simulink model "l512_devel_pps"  (R2012b)
settings: Solver=ode45  StartTime=0.0  StopTime=15000  RelTol=1e-3
undefined symbols (not defined in the file): sfp
libraries: xbsIndex_r4 x6414, casper_library_misc x268, casper_library_delays x134, xps_library x12, simulink x1, gavrt_library x1, xbsReplacements_r4 x1
(part 13 of 67)

== system l512_devel_pps/fft/f3/rms_mon_4b ==
  note: Value on vin
      | aligned with
      | first sample on
      | din captured
  note: Number of valid
      | data samples to
      | skip after trigger
      | before starting
      | capture
  note: Number of
      | bytes in
      | buffer and
      | done bit
  note: Offset in vector
      | from first element
      | captured, used
      | during circular capture
  note: ctrl:
      | bit0: Put a posedge here
      |         to enable a new capture.
      | bit1: ignore external trigger
      |         and trigger immediately.
      | bit2: ignore external write
      |         enable and capture on
      |         every FPGA clock.
      | bit3: continuously capture
      |         data until we get an
      |         external stop command.
  note: Delay start
      | of capture
  note: Generate stop
      | when in circular
      | capture mode
  din : Inport
  we : Inport  Port=2
  trig : Inport  Port=3
  add_del : xbsIndex_r4/Delay  rst=off  infoeditControl=Selection of Reset will increase slice count due to use of real FFs and instead of SRLs  en=off  latency=1  dbl_ovrd=off  reg_retiming=on  block_type=delay
      settings: block_version=11.4
  add_gen : Subsystem  AncestorBlock=casper_library_scopes/snapshot/add_gen  mask{counter_size=12+0+1, increment=1, nsamples=12, burst_size=0, use_dsp48=off}
      mask prompts: counter_size "Address counter size (2^?)"; increment "Address counter increment"; nsamples "Number of samples (2^?)"; burst_size "Burst size (2^?)"; use_dsp48 "dsp48 counter/s"
      mask init:
      | set_param(gcb,'LinkStatus','inactive');
      | if strcmp(use_dsp48,'on'),
      |     set_param([gcb,'/add_gen'],'implementation','DSP48');
      | else
      |     set_param([gcb,'/add_gen'],'implementation','Fabric');
      | end
  basic_ctrl : Subsystem  AncestorBlock=casper_library_scopes/snapshot/basic_ctrl  mask{dram=off, data_width=8}
      mask prompts: data_width "data width"
      mask init:
      | set_param(gcb,'LinkStatus','inactive');
      | set_param([gcb,'/dram_munge'], 'dram', dram);
  bram : Subsystem  Tag=xps:bram  AncestorBlock=xps_library/Shared BRAM  mask{arith_type=Unsigned, addr_width=12, data_width=8, reg_prim_output=on, reg_core_output=on, optimization=Minimum_Area, data_bin_pt=0, init_vals=[0:2^10-1], sample_rate=1}
      mask prompts: arith_type "Output Data Type"; addr_width "Address width"; data_width "Data Width"; reg_prim_output "Register Primitive Output"; reg_core_output "Register Core Output"; data_bin_pt "Data Binary Point"; init_vals "Initial values (simulation only)"; sample_rate "Sample rate"
      mask init:
      | shared_bram_mask;
      mask TypeOptions arith_type: Unsigned | Signed  (2's comp)
      mask TypeOptions data_width: 8 | 16 | 32 | 64 | 128
      mask TypeOptions optimization: Minimum_Area | Low_Power
  cast : xbsIndex_r4/Convert  gui_display_data_type=Fixed-point  arith_type=Unsigned  n_bits=8  bin_pt=0  float_type=Single  exp_bits=8  fraction_bits=24  quantization=Truncate  overflow=Wrap  en=off  latency=0  dbl_ovrd=off  pipeline=off  block_type=convert
      settings: block_version=11.4
  circular_capture : casper_library_misc/info_block  Tag=casper:info  info=off
  const0 : Constant  Value=0
  ctrl : Subsystem  Tag=xps:sw_reg  AncestorBlock=xps_library/software register  mask{numios=1, io_dir=From Processor, io_delay=0, sample_period=1, name1=reg, bitwidth1=32, arith_type1=Unsigned, bin_pt1=0}
      mask prompts: numios "Num I/Os"; io_dir "I/O direction"; io_delay "I/O delay"; sample_period "Sample period"; name1 "Name"; bitwidth1 "Bitwidth"; arith_type1 "Type"; bin_pt1 "Binary pt"
      mask init:
      | swreg_init(gcb);
      mask Callback numios: t = timer('StartDelay', 0.1); t.TimerFcn = {@swreg_cb, gcb}; start(t);
      mask TypeOptions io_dir: To Processor | From Processor
      mask Callback io_dir:
      | a = get_param(gcb, 'MaskEnables');
      | if strcmp(get_param(gcb, 'io_dir'), 'To Processor'),
      | a(4) = {'off'};
      | else
      | a(4) = {'on'};
      | end
      | set_param(gcb, 'MaskEnables', a);
      mask TypeOptions arith_type1: Unsigned | Signed  (2's comp) | Boolean
      mask Callback arith_type1:
      | a = get_param(gcb, 'MaskEnables');
      | if strcmp(get_param(gcb, 'arith_type1'), 'Boolean'),
      | set_param(gcb, 'bitwidth1', '1');
      | set_param(gcb, 'bin_pt1', '0');
      | a(6) = {'off'};
      | a(8) = {'off'};
      | else
      | a(6) = {'on'};
      | a(8) = {'on'};
      | end
      | set_param(gcb, 'MaskEnables', a);
  dat_del : xbsIndex_r4/Delay  rst=off  infoeditControl=Selection of Reset will increase slice count due to use of real FFs and instead of SRLs  en=off  latency=1  dbl_ovrd=off  reg_retiming=on  block_type=delay
      settings: block_version=11.4
  data_width : casper_library_misc/info_block  Tag=casper:info  info=8
  dram_clock : casper_library_misc/info_block  Tag=casper:info  info=200
  dram_dimm : casper_library_misc/info_block  Tag=casper:info  info=1
  extra_value : casper_library_misc/info_block  Tag=casper:info  info=off
  g_tr_en_cnt : Terminator
  gbram : Terminator
  gstatus : Terminator
  gval : Terminator
  length : casper_library_misc/info_block  Tag=casper:info  info=4096
  never : xbsIndex_r4/Constant  const=0  gui_display_data_type=Fixed-point  arith_type=Boolean  n_bits=16  bin_pt=14  preci_type=Single  exp_width=8  frac_width=24  explicit_period=on  period=1  equ=P=C  opselect=C  inp2=PCIN>>17  opr=+  inp1=P  carry=CIN  dbl_ovrd=off  block_type=constant
  ri : xbsIndex_r4/Reinterpret  force_arith_type=on  arith_type=Unsigned  force_bin_pt=on  bin_pt=0  block_type=reinterpret
      settings: infoedit="Changes signal type without altering the binary representation.   You can changed the signal between signed and unsigned, and relocate the binary point.<br><br>Hardware notes: In hardware this block costs nothing.<br><br>Example:  Suppose the input is 6 bits wide, signed, with 2 fractional bits, and the output is forced to unsigned with 0 fractional bits.  Then an input of -2.0 (1110.00 in binary 2's complement) becomes an output of 56 (111000 in binary)."
  start_offset : casper_library_misc/info_block  Tag=casper:info  info=off
  status : Subsystem  Tag=xps:sw_reg  AncestorBlock=xps_library/software register  mask{numios=1, io_dir=To Processor, io_delay=0, sample_period=1, name1=reg, bitwidth1=32, arith_type1=Unsigned, bin_pt1=0}
      mask prompts: numios "Num I/Os"; io_dir "I/O direction"; io_delay "I/O delay"; sample_period "Sample period"; name1 "Name"; bitwidth1 "Bitwidth"; arith_type1 "Type"; bin_pt1 "Binary pt"
      mask init:
      | swreg_init(gcb);
      mask Callback numios: t = timer('StartDelay', 0.1); t.TimerFcn = {@swreg_cb, gcb}; start(t);
      mask TypeOptions io_dir: To Processor | From Processor
      mask Callback io_dir:
      | a = get_param(gcb, 'MaskEnables');
      | if strcmp(get_param(gcb, 'io_dir'), 'To Processor'),
      | a(4) = {'off'};
      | else
      | a(4) = {'on'};
      | end
      | set_param(gcb, 'MaskEnables', a);
      mask TypeOptions arith_type1: Unsigned | Signed  (2's comp) | Boolean
      mask Callback arith_type1:
      | a = get_param(gcb, 'MaskEnables');
      | if strcmp(get_param(gcb, 'arith_type1'), 'Boolean'),
      | set_param(gcb, 'bitwidth1', '1');
      | set_param(gcb, 'bin_pt1', '0');
      | a(6) = {'off'};
      | a(8) = {'off'};
      | else
      | a(6) = {'on'};
      | a(8) = {'on'};
      | end
      | set_param(gcb, 'MaskEnables', a);
  storage : casper_library_misc/info_block  Tag=casper:info  info=bram
  use_dsp48 : casper_library_misc/info_block  Tag=casper:info  info=off
  vin_const : xbsIndex_r4/Constant  const=0  gui_display_data_type=Fixed-point  arith_type=Boolean  n_bits=16  bin_pt=14  preci_type=Single  exp_width=8  frac_width=24  explicit_period=on  period=1  equ=P=C  opselect=C  inp2=PCIN>>17  opr=+  inp1=P  carry=CIN  dbl_ovrd=off  block_type=constant
      settings: block_version=11.4
  we_del : xbsIndex_r4/Delay  rst=off  infoeditControl=Selection of Reset will increase slice count due to use of real FFs and instead of SRLs  en=off  latency=1  dbl_ovrd=off  reg_retiming=on  block_type=delay
      settings: block_version=11.4
  wires:
  bram/1(data_out) -> gbram/1
  we_del/1 -> bram/3(we)
  dat_del/1 -> bram/2(data_in)
  add_del/1 -> bram/1(addr)
  add_gen/4(we_o) -> we_del/1
  add_gen/3(dout) -> dat_del/1
  add_gen/2(add) -> add_del/1
  add_gen/6(en_cnt) -> g_tr_en_cnt/1
  add_gen/1(vout) -> gval/1
  vin_const/1 -> basic_ctrl/1(vin)
  status/1(sim_out) -> gstatus/1
  add_gen/5(status) -> status/1(out_reg)
  basic_ctrl/6(init) -> add_gen/6(init)
  basic_ctrl/5(stop) -> add_gen/5(cont)
  basic_ctrl/4(go) -> add_gen/4(go)
  basic_ctrl/3(we_o) -> add_gen/3(we)
  basic_ctrl/2(dout) -> add_gen/2(din)
  basic_ctrl/1(vout) -> add_gen/1(vin)
  ctrl/1(in_reg) -> basic_ctrl/5(ctrl)
  const0/1 -> ctrl/1(sim_reg)
  never/1 -> basic_ctrl/6(stopi)
  trig/1 -> basic_ctrl/4(trig)
  we/1 -> basic_ctrl/3(we)
  cast/1 -> basic_ctrl/2(din)
  ri/1 -> cast/1
  din/1 -> ri/1

== system l512_devel_pps/fft/f3/spec0 ==
  sync_in : Inport
  pps_in : Inport  Port=2
  d_in : Inport  Port=3
  bitsel : Inport  Port=4
  acc_len : Inport  Port=5
  Delay1 : xbsIndex_r4/Delay  rst=off  infoeditControl=Selection of Reset will increase slice count due to use of real FFs and instead of SRLs  en=off  latency=4  dbl_ovrd=off  reg_retiming=off  block_type=delay
  Delay2 : xbsIndex_r4/Delay  rst=off  infoeditControl=Selection of Reset will increase slice count due to use of real FFs and instead of SRLs  en=off  latency=2  dbl_ovrd=off  reg_retiming=off  block_type=delay
  Delay6 : xbsIndex_r4/Delay  rst=off  infoeditControl=Selection of Reset will increase slice count due to use of real FFs and instead of SRLs  en=off  latency=2  dbl_ovrd=off  reg_retiming=off  block_type=delay
  edge_detect2 : casper_library_misc/edge_detect  edge=Rising  polarity=Active High  x_in=[0 0.08 0.08 0.16 0.16 0.24 0.24 0.32 0.32 0.4]  y_in="[-1 -1  1  1  1  1  1  1  1  1]"  x_out=[0.6 0.68 0.68 0.76 0.76 0.84 0.84 0.92 0.92 1]  y_out="[-1 -1  1  1 -1 -1 -1 -1 -1 -1]"
  pipeline4 : Subsystem  AncestorBlock=casper_library_delays/pipeline  mask(pipeline){latency=1}
      mask help:
      | An explicitly laid-out delay line to avoid mapping to SRL16s
      | for use in pipelining to help achieve timing closure.
      mask init:
      | pipeline_init(gcb,'latency',latency);
      settings: AttributesFormatString=Latency = %<latency>
      mask Display:
      | port_label('input', 1, 'd');
      | port_label('output', 1, 'q');
      | disp(['Z^-', num2str(latency)]);
  pipeline5 : Subsystem  AncestorBlock=casper_library_delays/pipeline  mask(pipeline){latency=1}
      mask help:
      | An explicitly laid-out delay line to avoid mapping to SRL16s
      | for use in pipelining to help achieve timing closure.
      mask init:
      | pipeline_init(gcb,'latency',latency);
      settings: AttributesFormatString=Latency = %<latency>
      mask Display:
      | port_label('input', 1, 'd');
      | port_label('output', 1, 'q');
      | disp(['Z^-', num2str(latency)]);
  pipeline6 : Subsystem  AncestorBlock=casper_library_delays/pipeline  mask(pipeline){latency=1}
      mask help:
      | An explicitly laid-out delay line to avoid mapping to SRL16s
      | for use in pipelining to help achieve timing closure.
      mask init:
      | pipeline_init(gcb,'latency',latency);
      settings: AttributesFormatString=Latency = %<latency>
      mask Display:
      | port_label('input', 1, 'd');
      | port_label('output', 1, 'q');
      | disp(['Z^-', num2str(latency)]);
  power_dsp48e3 : casper_library_misc/power_dsp48e  bitwidth=18
  rq : Subsystem
  snap : Subsystem  mask{vec_bits=12}
      mask prompts: vec_bits "Vector length (2^N)"
  sync_delay : casper_library_delays/sync_delay  DelayLen=10
  vacc_pps : Subsystem  mask{n_fft=12}
      mask prompts: n_fft "Length of FFT (2^N)?"
  vacc_zeroer1 : Subsystem  mask{nbits=13, bw=16}
      mask prompts: nbits "FFT length (2^N)?"; bw "bitwidth in"
      mask help: FFT length is full length of FFT. The second half will be blanked.
  new_acc : Outport
  wires:
  vacc_pps/2(d_out) -> pipeline4/1(d)
  vacc_zeroer1/1(sync_out) -> vacc_pps/1(sync_in)
  sync_delay/1 -> vacc_pps/2(pps_in)
  pps_in/1 -> sync_delay/1
  power_dsp48e3/1 -> rq/2(d_in)
  pipeline6/1(q) -> edge_detect2/1
  bitsel/1 -> rq/3(bitsel)
  vacc_zeroer1/2(d_out) -> vacc_pps/4(d_in)
  d_in/1 -> power_dsp48e3/1
  sync_in/1 -> Delay1/1
  rq/2(d_out) -> vacc_zeroer1/2(d_in)
  Delay1/1 -> rq/1(sync_in)
  Delay6/1 -> snap/2(data_valid)
  acc_len/1 -> vacc_pps/3(acc_len)
  edge_detect2/1 -> snap/1(new_acc), new_acc/1
  pipeline4/1(q) -> Delay2/1
  Delay2/1 -> snap/3(xx_in)
  vacc_pps/1(valid_out) -> pipeline5/1(d), pipeline6/1(d)
  rq/1(sync_out) -> vacc_zeroer1/1(sync_in)
  pipeline5/1(q) -> Delay6/1

== system l512_devel_pps/fft/f3/spec1 ==
  sync_in : Inport
  pps_in : Inport  Port=2
  d_in : Inport  Port=3
  bitsel : Inport  Port=4
  acc_len : Inport  Port=5
  Delay1 : xbsIndex_r4/Delay  rst=off  infoeditControl=Selection of Reset will increase slice count due to use of real FFs and instead of SRLs  en=off  latency=4  dbl_ovrd=off  reg_retiming=off  block_type=delay
  Delay2 : xbsIndex_r4/Delay  rst=off  infoeditControl=Selection of Reset will increase slice count due to use of real FFs and instead of SRLs  en=off  latency=2  dbl_ovrd=off  reg_retiming=off  block_type=delay
  Delay6 : xbsIndex_r4/Delay  rst=off  infoeditControl=Selection of Reset will increase slice count due to use of real FFs and instead of SRLs  en=off  latency=2  dbl_ovrd=off  reg_retiming=off  block_type=delay
  edge_detect2 : casper_library_misc/edge_detect  edge=Rising  polarity=Active High  x_in=[0 0.08 0.08 0.16 0.16 0.24 0.24 0.32 0.32 0.4]  y_in="[-1 -1  1  1  1  1  1  1  1  1]"  x_out=[0.6 0.68 0.68 0.76 0.76 0.84 0.84 0.92 0.92 1]  y_out="[-1 -1  1  1 -1 -1 -1 -1 -1 -1]"
  pipeline4 : Subsystem  AncestorBlock=casper_library_delays/pipeline  mask(pipeline){latency=1}
      mask help:
      | An explicitly laid-out delay line to avoid mapping to SRL16s
      | for use in pipelining to help achieve timing closure.
      mask init:
      | pipeline_init(gcb,'latency',latency);
      settings: AttributesFormatString=Latency = %<latency>
      mask Display:
      | port_label('input', 1, 'd');
      | port_label('output', 1, 'q');
      | disp(['Z^-', num2str(latency)]);
  pipeline5 : Subsystem  AncestorBlock=casper_library_delays/pipeline  mask(pipeline){latency=1}
      mask help:
      | An explicitly laid-out delay line to avoid mapping to SRL16s
      | for use in pipelining to help achieve timing closure.
      mask init:
      | pipeline_init(gcb,'latency',latency);
      settings: AttributesFormatString=Latency = %<latency>
      mask Display:
      | port_label('input', 1, 'd');
      | port_label('output', 1, 'q');
      | disp(['Z^-', num2str(latency)]);
  pipeline6 : Subsystem  AncestorBlock=casper_library_delays/pipeline  mask(pipeline){latency=1}
      mask help:
      | An explicitly laid-out delay line to avoid mapping to SRL16s
      | for use in pipelining to help achieve timing closure.
      mask init:
      | pipeline_init(gcb,'latency',latency);
      settings: AttributesFormatString=Latency = %<latency>
      mask Display:
      | port_label('input', 1, 'd');
      | port_label('output', 1, 'q');
      | disp(['Z^-', num2str(latency)]);
  power_dsp48e3 : casper_library_misc/power_dsp48e  bitwidth=18
  rq : Subsystem
  snap : Subsystem  mask{vec_bits=12}
      mask prompts: vec_bits "Vector length (2^N)"
  sync_delay : casper_library_delays/sync_delay  DelayLen=10
  vacc_pps : Subsystem  mask{n_fft=12}
      mask prompts: n_fft "Length of FFT (2^N)?"
  vacc_zeroer1 : Subsystem  mask{nbits=13, bw=16}
      mask prompts: nbits "FFT length (2^N)?"; bw "bitwidth in"
      mask help: FFT length is full length of FFT. The second half will be blanked.
  new_acc : Outport
  wires:
  pipeline5/1(q) -> Delay6/1
  rq/1(sync_out) -> vacc_zeroer1/1(sync_in)
  vacc_pps/1(valid_out) -> pipeline6/1(d), pipeline5/1(d)
  Delay2/1 -> snap/3(xx_in)
  pipeline4/1(q) -> Delay2/1
  edge_detect2/1 -> new_acc/1, snap/1(new_acc)
  acc_len/1 -> vacc_pps/3(acc_len)
  Delay6/1 -> snap/2(data_valid)
  Delay1/1 -> rq/1(sync_in)
  rq/2(d_out) -> vacc_zeroer1/2(d_in)
  sync_in/1 -> Delay1/1
  d_in/1 -> power_dsp48e3/1
  vacc_zeroer1/2(d_out) -> vacc_pps/4(d_in)
  bitsel/1 -> rq/3(bitsel)
  pipeline6/1(q) -> edge_detect2/1
  power_dsp48e3/1 -> rq/2(d_in)
  pps_in/1 -> sync_delay/1
  sync_delay/1 -> vacc_pps/2(pps_in)
  vacc_zeroer1/1(sync_out) -> vacc_pps/1(sync_in)
  vacc_pps/2(d_out) -> pipeline4/1(d)

== system l512_devel_pps/fft/f3/spec2 ==
  sync_in : Inport
  pps_in : Inport  Port=2
  d_in : Inport  Port=3
  bitsel : Inport  Port=4
  acc_len : Inport  Port=5
  Delay1 : xbsIndex_r4/Delay  rst=off  infoeditControl=Selection of Reset will increase slice count due to use of real FFs and instead of SRLs  en=off  latency=4  dbl_ovrd=off  reg_retiming=off  block_type=delay
  Delay2 : xbsIndex_r4/Delay  rst=off  infoeditControl=Selection of Reset will increase slice count due to use of real FFs and instead of SRLs  en=off  latency=2  dbl_ovrd=off  reg_retiming=off  block_type=delay
  Delay6 : xbsIndex_r4/Delay  rst=off  infoeditControl=Selection of Reset will increase slice count due to use of real FFs and instead of SRLs  en=off  latency=2  dbl_ovrd=off  reg_retiming=off  block_type=delay
  edge_detect2 : casper_library_misc/edge_detect  edge=Rising  polarity=Active High  x_in=[0 0.08 0.08 0.16 0.16 0.24 0.24 0.32 0.32 0.4]  y_in="[-1 -1  1  1  1  1  1  1  1  1]"  x_out=[0.6 0.68 0.68 0.76 0.76 0.84 0.84 0.92 0.92 1]  y_out="[-1 -1  1  1 -1 -1 -1 -1 -1 -1]"
  pipeline4 : Subsystem  AncestorBlock=casper_library_delays/pipeline  mask(pipeline){latency=1}
      mask help:
      | An explicitly laid-out delay line to avoid mapping to SRL16s
      | for use in pipelining to help achieve timing closure.
      mask init:
      | pipeline_init(gcb,'latency',latency);
      settings: AttributesFormatString=Latency = %<latency>
      mask Display:
      | port_label('input', 1, 'd');
      | port_label('output', 1, 'q');
      | disp(['Z^-', num2str(latency)]);
  pipeline5 : Subsystem  AncestorBlock=casper_library_delays/pipeline  mask(pipeline){latency=1}
      mask help:
      | An explicitly laid-out delay line to avoid mapping to SRL16s
      | for use in pipelining to help achieve timing closure.
      mask init:
      | pipeline_init(gcb,'latency',latency);
      settings: AttributesFormatString=Latency = %<latency>
      mask Display:
      | port_label('input', 1, 'd');
      | port_label('output', 1, 'q');
      | disp(['Z^-', num2str(latency)]);
  pipeline6 : Subsystem  AncestorBlock=casper_library_delays/pipeline  mask(pipeline){latency=1}
      mask help:
      | An explicitly laid-out delay line to avoid mapping to SRL16s
      | for use in pipelining to help achieve timing closure.
      mask init:
      | pipeline_init(gcb,'latency',latency);
      settings: AttributesFormatString=Latency = %<latency>
      mask Display:
      | port_label('input', 1, 'd');
      | port_label('output', 1, 'q');
      | disp(['Z^-', num2str(latency)]);
  power_dsp48e3 : casper_library_misc/power_dsp48e  bitwidth=18
  rq : Subsystem
  snap : Subsystem  mask{vec_bits=12}
      mask prompts: vec_bits "Vector length (2^N)"
  sync_delay : casper_library_delays/sync_delay  DelayLen=10
  vacc_pps : Subsystem  mask{n_fft=12}
      mask prompts: n_fft "Length of FFT (2^N)?"
  vacc_zeroer1 : Subsystem  mask{nbits=13, bw=16}
      mask prompts: nbits "FFT length (2^N)?"; bw "bitwidth in"
      mask help: FFT length is full length of FFT. The second half will be blanked.
  new_acc : Outport
  wires:
  vacc_pps/2(d_out) -> pipeline4/1(d)
  vacc_zeroer1/1(sync_out) -> vacc_pps/1(sync_in)
  sync_delay/1 -> vacc_pps/2(pps_in)
  pps_in/1 -> sync_delay/1
  power_dsp48e3/1 -> rq/2(d_in)
  pipeline6/1(q) -> edge_detect2/1
  bitsel/1 -> rq/3(bitsel)
  vacc_zeroer1/2(d_out) -> vacc_pps/4(d_in)
  d_in/1 -> power_dsp48e3/1
  sync_in/1 -> Delay1/1
  rq/2(d_out) -> vacc_zeroer1/2(d_in)
  Delay1/1 -> rq/1(sync_in)
  Delay6/1 -> snap/2(data_valid)
  acc_len/1 -> vacc_pps/3(acc_len)
  edge_detect2/1 -> snap/1(new_acc), new_acc/1
  pipeline4/1(q) -> Delay2/1
  Delay2/1 -> snap/3(xx_in)
  vacc_pps/1(valid_out) -> pipeline5/1(d), pipeline6/1(d)
  rq/1(sync_out) -> vacc_zeroer1/1(sync_in)
  pipeline5/1(q) -> Delay6/1

== system l512_devel_pps/fft/f3/spec3 ==
  sync_in : Inport
  pps_in : Inport  Port=2
  d_in : Inport  Port=3
  bitsel : Inport  Port=4
  acc_len : Inport  Port=5
  Delay1 : xbsIndex_r4/Delay  rst=off  infoeditControl=Selection of Reset will increase slice count due to use of real FFs and instead of SRLs  en=off  latency=4  dbl_ovrd=off  reg_retiming=off  block_type=delay
  Delay2 : xbsIndex_r4/Delay  rst=off  infoeditControl=Selection of Reset will increase slice count due to use of real FFs and instead of SRLs  en=off  latency=2  dbl_ovrd=off  reg_retiming=off  block_type=delay
  Delay6 : xbsIndex_r4/Delay  rst=off  infoeditControl=Selection of Reset will increase slice count due to use of real FFs and instead of SRLs  en=off  latency=2  dbl_ovrd=off  reg_retiming=off  block_type=delay
  edge_detect2 : casper_library_misc/edge_detect  edge=Rising  polarity=Active High  x_in=[0 0.08 0.08 0.16 0.16 0.24 0.24 0.32 0.32 0.4]  y_in="[-1 -1  1  1  1  1  1  1  1  1]"  x_out=[0.6 0.68 0.68 0.76 0.76 0.84 0.84 0.92 0.92 1]  y_out="[-1 -1  1  1 -1 -1 -1 -1 -1 -1]"
  pipeline4 : Subsystem  AncestorBlock=casper_library_delays/pipeline  mask(pipeline){latency=1}
      mask help:
      | An explicitly laid-out delay line to avoid mapping to SRL16s
      | for use in pipelining to help achieve timing closure.
      mask init:
      | pipeline_init(gcb,'latency',latency);
      settings: AttributesFormatString=Latency = %<latency>
      mask Display:
      | port_label('input', 1, 'd');
      | port_label('output', 1, 'q');
      | disp(['Z^-', num2str(latency)]);
  pipeline5 : Subsystem  AncestorBlock=casper_library_delays/pipeline  mask(pipeline){latency=1}
      mask help:
      | An explicitly laid-out delay line to avoid mapping to SRL16s
      | for use in pipelining to help achieve timing closure.
      mask init:
      | pipeline_init(gcb,'latency',latency);
      settings: AttributesFormatString=Latency = %<latency>
      mask Display:
      | port_label('input', 1, 'd');
      | port_label('output', 1, 'q');
      | disp(['Z^-', num2str(latency)]);
  pipeline6 : Subsystem  AncestorBlock=casper_library_delays/pipeline  mask(pipeline){latency=1}
      mask help:
      | An explicitly laid-out delay line to avoid mapping to SRL16s
      | for use in pipelining to help achieve timing closure.
      mask init:
      | pipeline_init(gcb,'latency',latency);
      settings: AttributesFormatString=Latency = %<latency>
      mask Display:
      | port_label('input', 1, 'd');
      | port_label('output', 1, 'q');
      | disp(['Z^-', num2str(latency)]);
  power_dsp48e3 : casper_library_misc/power_dsp48e  bitwidth=18
  rq : Subsystem
  snap : Subsystem  mask{vec_bits=12}
      mask prompts: vec_bits "Vector length (2^N)"
  sync_delay : casper_library_delays/sync_delay  DelayLen=10
  vacc_pps : Subsystem  mask{n_fft=12}
      mask prompts: n_fft "Length of FFT (2^N)?"
  vacc_zeroer1 : Subsystem  mask{nbits=13, bw=16}
      mask prompts: nbits "FFT length (2^N)?"; bw "bitwidth in"
      mask help: FFT length is full length of FFT. The second half will be blanked.
  new_acc : Outport
  wires:
  pipeline5/1(q) -> Delay6/1
  rq/1(sync_out) -> vacc_zeroer1/1(sync_in)
  vacc_pps/1(valid_out) -> pipeline6/1(d), pipeline5/1(d)
  Delay2/1 -> snap/3(xx_in)
  pipeline4/1(q) -> Delay2/1
  edge_detect2/1 -> new_acc/1, snap/1(new_acc)
  acc_len/1 -> vacc_pps/3(acc_len)
  Delay6/1 -> snap/2(data_valid)
  Delay1/1 -> rq/1(sync_in)
  rq/2(d_out) -> vacc_zeroer1/2(d_in)
  sync_in/1 -> Delay1/1
  d_in/1 -> power_dsp48e3/1
  vacc_zeroer1/2(d_out) -> vacc_pps/4(d_in)
  bitsel/1 -> rq/3(bitsel)
  pipeline6/1(q) -> edge_detect2/1
  power_dsp48e3/1 -> rq/2(d_in)
  pps_in/1 -> sync_delay/1
  sync_delay/1 -> vacc_pps/2(pps_in)
  vacc_zeroer1/1(sync_out) -> vacc_pps/1(sync_in)
  vacc_pps/2(d_out) -> pipeline4/1(d)

== system l512_devel_pps/fft/f3/spec4 ==
  sync_in : Inport
  pps_in : Inport  Port=2
  d_in : Inport  Port=3
  bitsel : Inport  Port=4
  acc_len : Inport  Port=5
  Delay1 : xbsIndex_r4/Delay  rst=off  infoeditControl=Selection of Reset will increase slice count due to use of real FFs and instead of SRLs  en=off  latency=4  dbl_ovrd=off  reg_retiming=off  block_type=delay
  Delay2 : xbsIndex_r4/Delay  rst=off  infoeditControl=Selection of Reset will increase slice count due to use of real FFs and instead of SRLs  en=off  latency=2  dbl_ovrd=off  reg_retiming=off  block_type=delay
  Delay6 : xbsIndex_r4/Delay  rst=off  infoeditControl=Selection of Reset will increase slice count due to use of real FFs and instead of SRLs  en=off  latency=2  dbl_ovrd=off  reg_retiming=off  block_type=delay
  edge_detect2 : casper_library_misc/edge_detect  edge=Rising  polarity=Active High  x_in=[0 0.08 0.08 0.16 0.16 0.24 0.24 0.32 0.32 0.4]  y_in="[-1 -1  1  1  1  1  1  1  1  1]"  x_out=[0.6 0.68 0.68 0.76 0.76 0.84 0.84 0.92 0.92 1]  y_out="[-1 -1  1  1 -1 -1 -1 -1 -1 -1]"
  pipeline4 : Subsystem  AncestorBlock=casper_library_delays/pipeline  mask(pipeline){latency=1}
      mask help:
      | An explicitly laid-out delay line to avoid mapping to SRL16s
      | for use in pipelining to help achieve timing closure.
      mask init:
      | pipeline_init(gcb,'latency',latency);
      settings: AttributesFormatString=Latency = %<latency>
      mask Display:
      | port_label('input', 1, 'd');
      | port_label('output', 1, 'q');
      | disp(['Z^-', num2str(latency)]);
  pipeline5 : Subsystem  AncestorBlock=casper_library_delays/pipeline  mask(pipeline){latency=1}
      mask help:
      | An explicitly laid-out delay line to avoid mapping to SRL16s
      | for use in pipelining to help achieve timing closure.
      mask init:
      | pipeline_init(gcb,'latency',latency);
      settings: AttributesFormatString=Latency = %<latency>
      mask Display:
      | port_label('input', 1, 'd');
      | port_label('output', 1, 'q');
      | disp(['Z^-', num2str(latency)]);
  pipeline6 : Subsystem  AncestorBlock=casper_library_delays/pipeline  mask(pipeline){latency=1}
      mask help:
      | An explicitly laid-out delay line to avoid mapping to SRL16s
      | for use in pipelining to help achieve timing closure.
      mask init:
      | pipeline_init(gcb,'latency',latency);
      settings: AttributesFormatString=Latency = %<latency>
      mask Display:
      | port_label('input', 1, 'd');
      | port_label('output', 1, 'q');
      | disp(['Z^-', num2str(latency)]);
  power_dsp48e3 : casper_library_misc/power_dsp48e  bitwidth=18
  rq : Subsystem
  snap : Subsystem  mask{vec_bits=12}
      mask prompts: vec_bits "Vector length (2^N)"
  sync_delay : casper_library_delays/sync_delay  DelayLen=10
  vacc_pps : Subsystem  mask{n_fft=12}
      mask prompts: n_fft "Length of FFT (2^N)?"
  vacc_zeroer1 : Subsystem  mask{nbits=13, bw=16}
      mask prompts: nbits "FFT length (2^N)?"; bw "bitwidth in"
      mask help: FFT length is full length of FFT. The second half will be blanked.
  new_acc : Outport
  wires:
  vacc_pps/2(d_out) -> pipeline4/1(d)
  vacc_zeroer1/1(sync_out) -> vacc_pps/1(sync_in)
  sync_delay/1 -> vacc_pps/2(pps_in)
  pps_in/1 -> sync_delay/1
  power_dsp48e3/1 -> rq/2(d_in)
  pipeline6/1(q) -> edge_detect2/1
  bitsel/1 -> rq/3(bitsel)
  vacc_zeroer1/2(d_out) -> vacc_pps/4(d_in)
  d_in/1 -> power_dsp48e3/1
  sync_in/1 -> Delay1/1
  rq/2(d_out) -> vacc_zeroer1/2(d_in)
  Delay1/1 -> rq/1(sync_in)
  Delay6/1 -> snap/2(data_valid)
  acc_len/1 -> vacc_pps/3(acc_len)
  edge_detect2/1 -> snap/1(new_acc), new_acc/1
  pipeline4/1(q) -> Delay2/1
  Delay2/1 -> snap/3(xx_in)
  vacc_pps/1(valid_out) -> pipeline5/1(d), pipeline6/1(d)
  rq/1(sync_out) -> vacc_zeroer1/1(sync_in)
  pipeline5/1(q) -> Delay6/1

== system l512_devel_pps/fft/f3/spec5 ==
  sync_in : Inport
  pps_in : Inport  Port=2
  d_in : Inport  Port=3
  bitsel : Inport  Port=4
  acc_len : Inport  Port=5
  Delay1 : xbsIndex_r4/Delay  rst=off  infoeditControl=Selection of Reset will increase slice count due to use of real FFs and instead of SRLs  en=off  latency=4  dbl_ovrd=off  reg_retiming=off  block_type=delay
  Delay2 : xbsIndex_r4/Delay  rst=off  infoeditControl=Selection of Reset will increase slice count due to use of real FFs and instead of SRLs  en=off  latency=2  dbl_ovrd=off  reg_retiming=off  block_type=delay
  Delay6 : xbsIndex_r4/Delay  rst=off  infoeditControl=Selection of Reset will increase slice count due to use of real FFs and instead of SRLs  en=off  latency=2  dbl_ovrd=off  reg_retiming=off  block_type=delay
  edge_detect2 : casper_library_misc/edge_detect  edge=Rising  polarity=Active High  x_in=[0 0.08 0.08 0.16 0.16 0.24 0.24 0.32 0.32 0.4]  y_in="[-1 -1  1  1  1  1  1  1  1  1]"  x_out=[0.6 0.68 0.68 0.76 0.76 0.84 0.84 0.92 0.92 1]  y_out="[-1 -1  1  1 -1 -1 -1 -1 -1 -1]"
  pipeline4 : Subsystem  AncestorBlock=casper_library_delays/pipeline  mask(pipeline){latency=1}
      mask help:
      | An explicitly laid-out delay line to avoid mapping to SRL16s
      | for use in pipelining to help achieve timing closure.
      mask init:
      | pipeline_init(gcb,'latency',latency);
      settings: AttributesFormatString=Latency = %<latency>
      mask Display:
      | port_label('input', 1, 'd');
      | port_label('output', 1, 'q');
      | disp(['Z^-', num2str(latency)]);
  pipeline5 : Subsystem  AncestorBlock=casper_library_delays/pipeline  mask(pipeline){latency=1}
      mask help:
      | An explicitly laid-out delay line to avoid mapping to SRL16s
      | for use in pipelining to help achieve timing closure.
      mask init:
      | pipeline_init(gcb,'latency',latency);
      settings: AttributesFormatString=Latency = %<latency>
      mask Display:
      | port_label('input', 1, 'd');
      | port_label('output', 1, 'q');
      | disp(['Z^-', num2str(latency)]);
  pipeline6 : Subsystem  AncestorBlock=casper_library_delays/pipeline  mask(pipeline){latency=1}
      mask help:
      | An explicitly laid-out delay line to avoid mapping to SRL16s
      | for use in pipelining to help achieve timing closure.
      mask init:
      | pipeline_init(gcb,'latency',latency);
      settings: AttributesFormatString=Latency = %<latency>
      mask Display:
      | port_label('input', 1, 'd');
      | port_label('output', 1, 'q');
      | disp(['Z^-', num2str(latency)]);
  power_dsp48e3 : casper_library_misc/power_dsp48e  bitwidth=18
  rq : Subsystem
  snap : Subsystem  mask{vec_bits=12}
      mask prompts: vec_bits "Vector length (2^N)"
  sync_delay : casper_library_delays/sync_delay  DelayLen=10
  vacc_pps : Subsystem  mask{n_fft=12}
      mask prompts: n_fft "Length of FFT (2^N)?"
  vacc_zeroer1 : Subsystem  mask{nbits=13, bw=16}
      mask prompts: nbits "FFT length (2^N)?"; bw "bitwidth in"
      mask help: FFT length is full length of FFT. The second half will be blanked.
  new_acc : Outport
  wires:
  pipeline5/1(q) -> Delay6/1
  rq/1(sync_out) -> vacc_zeroer1/1(sync_in)
  vacc_pps/1(valid_out) -> pipeline6/1(d), pipeline5/1(d)
  Delay2/1 -> snap/3(xx_in)
  pipeline4/1(q) -> Delay2/1
  edge_detect2/1 -> new_acc/1, snap/1(new_acc)
  acc_len/1 -> vacc_pps/3(acc_len)
  Delay6/1 -> snap/2(data_valid)
  Delay1/1 -> rq/1(sync_in)
  rq/2(d_out) -> vacc_zeroer1/2(d_in)
  sync_in/1 -> Delay1/1
  d_in/1 -> power_dsp48e3/1
  vacc_zeroer1/2(d_out) -> vacc_pps/4(d_in)
  bitsel/1 -> rq/3(bitsel)
  pipeline6/1(q) -> edge_detect2/1
  power_dsp48e3/1 -> rq/2(d_in)
  pps_in/1 -> sync_delay/1
  sync_delay/1 -> vacc_pps/2(pps_in)
  vacc_zeroer1/1(sync_out) -> vacc_pps/1(sync_in)
  vacc_pps/2(d_out) -> pipeline4/1(d)

== system l512_devel_pps/fft/f3/spec6 ==
  sync_in : Inport
  pps_in : Inport  Port=2
  d_in : Inport  Port=3
  bitsel : Inport  Port=4
  acc_len : Inport  Port=5
  Delay1 : xbsIndex_r4/Delay  rst=off  infoeditControl=Selection of Reset will increase slice count due to use of real FFs and instead of SRLs  en=off  latency=4  dbl_ovrd=off  reg_retiming=off  block_type=delay
  Delay2 : xbsIndex_r4/Delay  rst=off  infoeditControl=Selection of Reset will increase slice count due to use of real FFs and instead of SRLs  en=off  latency=2  dbl_ovrd=off  reg_retiming=off  block_type=delay
  Delay6 : xbsIndex_r4/Delay  rst=off  infoeditControl=Selection of Reset will increase slice count due to use of real FFs and instead of SRLs  en=off  latency=2  dbl_ovrd=off  reg_retiming=off  block_type=delay
  edge_detect2 : casper_library_misc/edge_detect  edge=Rising  polarity=Active High  x_in=[0 0.08 0.08 0.16 0.16 0.24 0.24 0.32 0.32 0.4]  y_in="[-1 -1  1  1  1  1  1  1  1  1]"  x_out=[0.6 0.68 0.68 0.76 0.76 0.84 0.84 0.92 0.92 1]  y_out="[-1 -1  1  1 -1 -1 -1 -1 -1 -1]"
  pipeline4 : Subsystem  AncestorBlock=casper_library_delays/pipeline  mask(pipeline){latency=1}
      mask help:
      | An explicitly laid-out delay line to avoid mapping to SRL16s
      | for use in pipelining to help achieve timing closure.
      mask init:
      | pipeline_init(gcb,'latency',latency);
      settings: AttributesFormatString=Latency = %<latency>
      mask Display:
      | port_label('input', 1, 'd');
      | port_label('output', 1, 'q');
      | disp(['Z^-', num2str(latency)]);
  pipeline5 : Subsystem  AncestorBlock=casper_library_delays/pipeline  mask(pipeline){latency=1}
      mask help:
      | An explicitly laid-out delay line to avoid mapping to SRL16s
      | for use in pipelining to help achieve timing closure.
      mask init:
      | pipeline_init(gcb,'latency',latency);
      settings: AttributesFormatString=Latency = %<latency>
      mask Display:
      | port_label('input', 1, 'd');
      | port_label('output', 1, 'q');
      | disp(['Z^-', num2str(latency)]);
  pipeline6 : Subsystem  AncestorBlock=casper_library_delays/pipeline  mask(pipeline){latency=1}
      mask help:
      | An explicitly laid-out delay line to avoid mapping to SRL16s
      | for use in pipelining to help achieve timing closure.
      mask init:
      | pipeline_init(gcb,'latency',latency);
      settings: AttributesFormatString=Latency = %<latency>
      mask Display:
      | port_label('input', 1, 'd');
      | port_label('output', 1, 'q');
      | disp(['Z^-', num2str(latency)]);
  power_dsp48e3 : casper_library_misc/power_dsp48e  bitwidth=18
  rq : Subsystem
  snap : Subsystem  mask{vec_bits=12}
      mask prompts: vec_bits "Vector length (2^N)"
  sync_delay : casper_library_delays/sync_delay  DelayLen=10
  vacc_pps : Subsystem  mask{n_fft=12}
      mask prompts: n_fft "Length of FFT (2^N)?"
  vacc_zeroer1 : Subsystem  mask{nbits=13, bw=16}
      mask prompts: nbits "FFT length (2^N)?"; bw "bitwidth in"
      mask help: FFT length is full length of FFT. The second half will be blanked.
  new_acc : Outport
  wires:
  vacc_pps/2(d_out) -> pipeline4/1(d)
  vacc_zeroer1/1(sync_out) -> vacc_pps/1(sync_in)
  sync_delay/1 -> vacc_pps/2(pps_in)
  pps_in/1 -> sync_delay/1
  power_dsp48e3/1 -> rq/2(d_in)
  pipeline6/1(q) -> edge_detect2/1
  bitsel/1 -> rq/3(bitsel)
  vacc_zeroer1/2(d_out) -> vacc_pps/4(d_in)
  d_in/1 -> power_dsp48e3/1
  sync_in/1 -> Delay1/1
  rq/2(d_out) -> vacc_zeroer1/2(d_in)
  Delay1/1 -> rq/1(sync_in)
  Delay6/1 -> snap/2(data_valid)
  acc_len/1 -> vacc_pps/3(acc_len)
  edge_detect2/1 -> snap/1(new_acc), new_acc/1
  pipeline4/1(q) -> Delay2/1
  Delay2/1 -> snap/3(xx_in)
  vacc_pps/1(valid_out) -> pipeline5/1(d), pipeline6/1(d)
  rq/1(sync_out) -> vacc_zeroer1/1(sync_in)
  pipeline5/1(q) -> Delay6/1

== system l512_devel_pps/fft/f3/spec7 ==
  sync_in : Inport
  pps_in : Inport  Port=2
  d_in : Inport  Port=3
  bitsel : Inport  Port=4
  acc_len : Inport  Port=5
  Delay1 : xbsIndex_r4/Delay  rst=off  infoeditControl=Selection of Reset will increase slice count due to use of real FFs and instead of SRLs  en=off  latency=4  dbl_ovrd=off  reg_retiming=off  block_type=delay
  Delay2 : xbsIndex_r4/Delay  rst=off  infoeditControl=Selection of Reset will increase slice count due to use of real FFs and instead of SRLs  en=off  latency=2  dbl_ovrd=off  reg_retiming=off  block_type=delay
  Delay6 : xbsIndex_r4/Delay  rst=off  infoeditControl=Selection of Reset will increase slice count due to use of real FFs and instead of SRLs  en=off  latency=2  dbl_ovrd=off  reg_retiming=off  block_type=delay
  edge_detect2 : casper_library_misc/edge_detect  edge=Rising  polarity=Active High  x_in=[0 0.08 0.08 0.16 0.16 0.24 0.24 0.32 0.32 0.4]  y_in="[-1 -1  1  1  1  1  1  1  1  1]"  x_out=[0.6 0.68 0.68 0.76 0.76 0.84 0.84 0.92 0.92 1]  y_out="[-1 -1  1  1 -1 -1 -1 -1 -1 -1]"
  pipeline4 : Subsystem  AncestorBlock=casper_library_delays/pipeline  mask(pipeline){latency=1}
      mask help:
      | An explicitly laid-out delay line to avoid mapping to SRL16s
      | for use in pipelining to help achieve timing closure.
      mask init:
      | pipeline_init(gcb,'latency',latency);
      settings: AttributesFormatString=Latency = %<latency>
      mask Display:
      | port_label('input', 1, 'd');
      | port_label('output', 1, 'q');
      | disp(['Z^-', num2str(latency)]);
  pipeline5 : Subsystem  AncestorBlock=casper_library_delays/pipeline  mask(pipeline){latency=1}
      mask help:
      | An explicitly laid-out delay line to avoid mapping to SRL16s
      | for use in pipelining to help achieve timing closure.
      mask init:
      | pipeline_init(gcb,'latency',latency);
      settings: AttributesFormatString=Latency = %<latency>
      mask Display:
      | port_label('input', 1, 'd');
      | port_label('output', 1, 'q');
      | disp(['Z^-', num2str(latency)]);
  pipeline6 : Subsystem  AncestorBlock=casper_library_delays/pipeline  mask(pipeline){latency=1}
      mask help:
      | An explicitly laid-out delay line to avoid mapping to SRL16s
      | for use in pipelining to help achieve timing closure.
      mask init:
      | pipeline_init(gcb,'latency',latency);
      settings: AttributesFormatString=Latency = %<latency>
      mask Display:
      | port_label('input', 1, 'd');
      | port_label('output', 1, 'q');
      | disp(['Z^-', num2str(latency)]);
  power_dsp48e3 : casper_library_misc/power_dsp48e  bitwidth=18
  rq : Subsystem
  snap : Subsystem  mask{vec_bits=12}
      mask prompts: vec_bits "Vector length (2^N)"
  sync_delay : casper_library_delays/sync_delay  DelayLen=10
  vacc_pps : Subsystem  mask{n_fft=12}
      mask prompts: n_fft "Length of FFT (2^N)?"
  vacc_zeroer1 : Subsystem  mask{nbits=13, bw=16}
      mask prompts: nbits "FFT length (2^N)?"; bw "bitwidth in"
      mask help: FFT length is full length of FFT. The second half will be blanked.
  new_acc : Outport
  wires:
  pipeline5/1(q) -> Delay6/1
  rq/1(sync_out) -> vacc_zeroer1/1(sync_in)
  vacc_pps/1(valid_out) -> pipeline6/1(d), pipeline5/1(d)
  Delay2/1 -> snap/3(xx_in)
  pipeline4/1(q) -> Delay2/1
  edge_detect2/1 -> new_acc/1, snap/1(new_acc)
  acc_len/1 -> vacc_pps/3(acc_len)
  Delay6/1 -> snap/2(data_valid)
  Delay1/1 -> rq/1(sync_in)
  rq/2(d_out) -> vacc_zeroer1/2(d_in)
  sync_in/1 -> Delay1/1
  d_in/1 -> power_dsp48e3/1
  vacc_zeroer1/2(d_out) -> vacc_pps/4(d_in)
  bitsel/1 -> rq/3(bitsel)
  pipeline6/1(q) -> edge_detect2/1
  power_dsp48e3/1 -> rq/2(d_in)
  pps_in/1 -> sync_delay/1
  sync_delay/1 -> vacc_pps/2(pps_in)
  vacc_zeroer1/1(sync_out) -> vacc_pps/1(sync_in)
  vacc_pps/2(d_out) -> pipeline4/1(d)

== system l512_devel_pps/fft/f4/acc_cnt ==
  out_reg : Inport
  cast_gw : xbsIndex_r4/Convert  gui_display_data_type=Fixed-point  arith_type=Unsigned  n_bits=32  bin_pt=0  float_type=Single  exp_bits=8  fraction_bits=24  quantization=Truncate  overflow=Wrap  en=off  latency=0  dbl_ovrd=off  pipeline=off  block_type=convert
  io_delay : xbsIndex_r4/Delay  rst=off  infoeditControl=Selection of Reset will increase slice count due to use of real FFs and instead of SRLs  en=off  latency=0  dbl_ovrd=off  reg_retiming=on  block_type=delay
  l512_devel_pps_fft_f4_acc_cnt_user_data_in : xbsIndex_r4/Gateway Out  inherit_from_input=off  hdl_port=on  timing_constraint=None  locs_specified=off  LOCs={}  UseAsDAC=off  DACChannel='1'  block_type=gatewayout
  reint1 : xbsIndex_r4/Reinterpret  force_arith_type=on  arith_type=Unsigned  force_bin_pt=on  bin_pt=0  block_type=reinterpret
  sim_out : Outport
  wires:
  io_delay/1 -> cast_gw/1
  cast_gw/1 -> l512_devel_pps_fft_f4_acc_cnt_user_data_in/1
  l512_devel_pps_fft_f4_acc_cnt_user_data_in/1 -> sim_out/1
  out_reg/1 -> reint1/1
  reint1/1 -> io_delay/1

== system l512_devel_pps/fft/f4/acc_len ==
  sim_reg : Inport
  io_delay : xbsIndex_r4/Delay  rst=off  infoeditControl=Selection of Reset will increase slice count due to use of real FFs and instead of SRLs  en=off  latency=0  dbl_ovrd=off  reg_retiming=on  block_type=delay
  l512_devel_pps_fft_f4_acc_len_user_data_out : xbsIndex_r4/Gateway In  gui_display_data_type=Fixed-point  arith_type=Unsigned  n_bits=32  bin_pt=0  preci_type=Single  exp_width=8  frac_width=24  quantization="Round  (unbiased: +/- Inf)"  overflow=Saturate  period=1  dbl_ovrd=off  timing_constraint=None  locs_specified=off  LOCs={}  UseAsADC=off  ADCChannel='1'  inherit_from_input=off  hdl_port=on  block_type=gatewayin
  reint1 : xbsIndex_r4/Reinterpret  force_arith_type=on  arith_type=Unsigned  force_bin_pt=on  bin_pt=0  block_type=reinterpret
  slice_reg : xbsIndex_r4/Slice  nbits=32  boolean_output=off  mode=Lower Bit Location + Width  bit1=0  base1=MSB of Input  bit0=0  base0=LSB of Input  dbl_ovrd=off  block_type=slice
  in_reg : Outport
  wires:
  l512_devel_pps_fft_f4_acc_len_user_data_out/1 -> io_delay/1
  sim_reg/1 -> l512_devel_pps_fft_f4_acc_len_user_data_out/1
  io_delay/1 -> slice_reg/1
  slice_reg/1 -> reint1/1
  reint1/1 -> in_reg/1

== system l512_devel_pps/fft/f4/bitsel ==
  sim_reg : Inport
  io_delay : xbsIndex_r4/Delay  rst=off  infoeditControl=Selection of Reset will increase slice count due to use of real FFs and instead of SRLs  en=off  latency=0  dbl_ovrd=off  reg_retiming=on  block_type=delay
  l512_devel_pps_fft_f4_bitsel_user_data_out : xbsIndex_r4/Gateway In  gui_display_data_type=Fixed-point  arith_type=Unsigned  n_bits=32  bin_pt=0  preci_type=Single  exp_width=8  frac_width=24  quantization="Round  (unbiased: +/- Inf)"  overflow=Saturate  period=1  dbl_ovrd=off  timing_constraint=None  locs_specified=off  LOCs={}  UseAsADC=off  ADCChannel='1'  inherit_from_input=off  hdl_port=on  block_type=gatewayin
  reint1 : xbsIndex_r4/Reinterpret  force_arith_type=on  arith_type=Unsigned  force_bin_pt=on  bin_pt=0  block_type=reinterpret
  slice_reg : xbsIndex_r4/Slice  nbits=32  boolean_output=off  mode=Lower Bit Location + Width  bit1=0  base1=MSB of Input  bit0=0  base0=LSB of Input  dbl_ovrd=off  block_type=slice
  in_reg : Outport
  wires:
  l512_devel_pps_fft_f4_bitsel_user_data_out/1 -> io_delay/1
  sim_reg/1 -> l512_devel_pps_fft_f4_bitsel_user_data_out/1
  io_delay/1 -> slice_reg/1
  slice_reg/1 -> reint1/1
  reint1/1 -> in_reg/1

== system l512_devel_pps/fft/f4/cg ==
  sync : Inport
  Delay1 : xbsIndex_r4/Delay  rst=off  infoeditControl=Selection of Reset will increase slice count due to use of real FFs and instead of SRLs  en=off  latency=4  dbl_ovrd=off  reg_retiming=off  block_type=delay
  Delay2 : xbsIndex_r4/Delay  rst=off  infoeditControl=Selection of Reset will increase slice count due to use of real FFs and instead of SRLs  en=off  latency=3  dbl_ovrd=off  reg_retiming=off  block_type=delay
  bpass : Subsystem
  sync_out : Outport
  coeffs_out : Outport  Port=2
  wires:
  Delay2/1 -> sync_out/1
  Delay1/1 -> Delay2/1
  sync/1 -> bpass/1(rst), Delay1/1
  bpass/1(coeffs_out) -> coeffs_out/1

== system l512_devel_pps/fft/f4/fft_shift ==
  sim_reg : Inport
  io_delay : xbsIndex_r4/Delay  rst=off  infoeditControl=Selection of Reset will increase slice count due to use of real FFs and instead of SRLs  en=off  latency=0  dbl_ovrd=off  reg_retiming=on  block_type=delay
  l512_devel_pps_fft_f4_fft_shift_user_data_out : xbsIndex_r4/Gateway In  gui_display_data_type=Fixed-point  arith_type=Unsigned  n_bits=32  bin_pt=0  preci_type=Single  exp_width=8  frac_width=24  quantization="Round  (unbiased: +/- Inf)"  overflow=Saturate  period=1  dbl_ovrd=off  timing_constraint=None  locs_specified=off  LOCs={}  UseAsADC=off  ADCChannel='1'  inherit_from_input=off  hdl_port=on  block_type=gatewayin
  reint1 : xbsIndex_r4/Reinterpret  force_arith_type=on  arith_type=Unsigned  force_bin_pt=on  bin_pt=0  block_type=reinterpret
  slice_reg : xbsIndex_r4/Slice  nbits=32  boolean_output=off  mode=Lower Bit Location + Width  bit1=0  base1=MSB of Input  bit0=0  base0=LSB of Input  dbl_ovrd=off  block_type=slice
  in_reg : Outport
  wires:
  l512_devel_pps_fft_f4_fft_shift_user_data_out/1 -> io_delay/1
  sim_reg/1 -> l512_devel_pps_fft_f4_fft_shift_user_data_out/1
  io_delay/1 -> slice_reg/1
  slice_reg/1 -> reint1/1
  reint1/1 -> in_reg/1

== system l512_devel_pps/fft/f4/pipeline ==
  d : Inport
  Register0 : xbsIndex_r4/Register  init=0  rst=off  en=off  dbl_ovrd=off  block_type=register
      settings: block_version=11.4
  q : Outport
  wires:
  Register0/1 -> q/1
  d/1 -> Register0/1

== system l512_devel_pps/fft/f4/pipeline1 ==
  d : Inport
  Register0 : xbsIndex_r4/Register  init=0  rst=off  en=off  dbl_ovrd=off  block_type=register
      settings: block_version=11.4
  q : Outport
  wires:
  Register0/1 -> q/1
  d/1 -> Register0/1

== system l512_devel_pps/fft/f4/pipeline2 ==
  d : Inport
  Register0 : xbsIndex_r4/Register  init=0  rst=off  en=off  dbl_ovrd=off  block_type=register
      settings: block_version=11.4
  q : Outport
  wires:
  d/1 -> Register0/1
  Register0/1 -> q/1

== system l512_devel_pps/fft/f4/pipeline3 ==
  d : Inport
  Register{0..3} (4 alike) : xbsIndex_r4/Register  init=0  rst=off  en=off  dbl_ovrd=off  block_type=register
      Register0 settings: block_version=11.4
  q : Outport
  wires:
  Register0/1 -> Register1/1
  Register1/1 -> Register2/1
  Register2/1 -> Register3/1
  d/1 -> Register0/1
  Register3/1 -> q/1

== system l512_devel_pps/fft/f4/pipeline45 ==
  d : Inport
  Register0 : xbsIndex_r4/Register  init=0  rst=off  en=off  dbl_ovrd=off  block_type=register
      settings: block_version=11.4
  q : Outport
  wires:
  Register0/1 -> q/1
  d/1 -> Register0/1

== system l512_devel_pps/fft/f4/pipeline8 ==
  d : Inport
  Register0 : xbsIndex_r4/Register  init=0  rst=off  en=off  dbl_ovrd=off  block_type=register
      settings: block_version=11.4
  q : Outport
  wires:
  d/1 -> Register0/1
  Register0/1 -> q/1
